simulink subsystem "observer_disc"  (R2023b)
settings: Solver=VariableStepAuto  StartTime=0.0  StopTime=10.0  RelTol=1e-3
values from neighbouring files (symbols this model uses):
  Ad = sysd.A    [sim_digitalcontrol.m]
  Bd = sysd.B    [sim_digitalcontrol.m]
  Cd = sysd.C    [sim_digitalcontrol.m]
  Dd = sysd.D    [sim_digitalcontrol.m]
  L = place(Adc', Cdc', obs_poles)'    [sim_digitalcontrol.m]
settings Model: Creator=kaitlin  LastModifiedBy=kaitlin

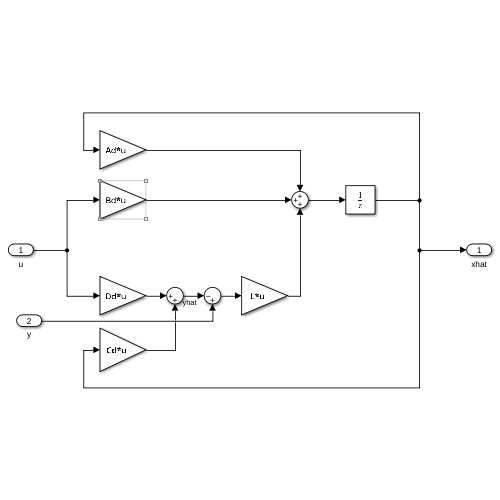
[thumbnail: Simulink's stored preview of the top-level diagram]
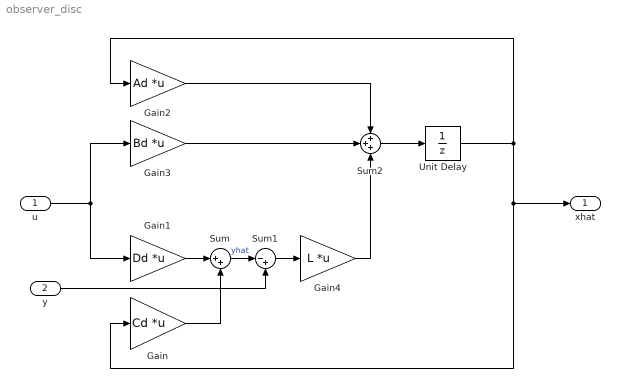
== system observer_disc ==
  u : Inport
  y : Inport  Port=2
  Gain : Gain  Gain=Cd  Multiplication=Matrix(K*u)
  Gain1 : Gain  Gain=Dd  Multiplication=Matrix(K*u)
  Gain2 : Gain  Gain=Ad  Multiplication=Matrix(K*u)
  Gain3 : Gain  Gain=Bd  Multiplication=Matrix(K*u)
  Gain4 : Gain  Gain=L  Multiplication=Matrix(K*u)
  Sum : Sum  Inputs=|++
  Sum1 : Sum  Inputs=|-+
  Sum2 : Sum  Inputs=+++
  Unit Delay : UnitDelay  SampleTime=-1  HasFrameUpgradeWarning=on
  xhat : Outport
  wires:
  Gain3/1 -> Sum2/2
  Gain4/1 -> Sum2/3
  u/1 -> Gain3/1, Gain1/1
  Sum2/1 -> Unit Delay/1
  Sum1/1 -> Gain4/1
  Gain/1 -> Sum/2
  Gain1/1 -> Sum/1
  Sum/1 -> Sum1/1  "yhat"
  y/1 -> Sum1/2
  Unit Delay/1 -> Gain/1, xhat/1, Gain2/1
  Gain2/1 -> Sum2/1
